simulink model "HIL_test"  (Simulink 7.5)
settings: Solver=FixedStepDiscrete  SolverMode=SingleTasking  StartTime=0.0  StopTime=10.0  FixedStep=0.01  RelTol=1e-3
undefined symbols (not defined in the file): enableHil, Function_Update, getSensorData, Init_onlyOnce, Init_Reset, initUart2, processNewCommData, y1
libraries: dsPICdrivers x7
settings Model: Creator=Bryant  LastModifiedBy=Bryant
settings OptimizationCC: OptimizeModelRefInitCode=on  LifeSpan=1
settings HardwareCC: ProdBitPerInt=16  ProdEndianess=LittleEndian  ProdWordSize=16  ProdHWDeviceType=16-bit Generic
settings RTWCC: SystemTargetFile=dspic.tlc  MakeCommand=make_CreateMPLAB  TemplateMakefile=dspic_pic30_gcc.tmf  PostCodeGenCommand=dsPIC_Compile()  Description=Embedded Target for Microchip dsPIC (real-time)  ProcessScript=dspic_make_rtw_hook
settings RTWCC: CustomSource=|
  | ../clib/circBuffer.c
  | ../clib/commProtocol.c
  | ../clib/uart2.c
settings CodeAppCC: IgnoreCustomStorageClasses=off
settings STFCustomTargetCC: IncludeMdlTerminateFcn=off  CombineOutputUpdateFcns=on  SuppressErrorStatus=on  ERTCustomFileBanners=on  SupportContinuousTime=off  SupportNonInlinedSFcns=off  SystemTargetFile=dspic.tlc
settings ERTTargetCC: MultiwordLength=2048  ParMdlRefBuildCompliant=off  CompOptLevelCompliant=off  IncludeMdlTerminateFcn=off  SuppressErrorStatus=on  ERTFirstTimeCompliant=off  ModelStepFunctionPrototypeControlCompliant=off  CPPClassGenCompliant=off  ExtModeMexFile=ext_serial_win32_comm  InlinedParameterPlacement=NonHierarchical  ERTSrcFileBannerTemplate=dsPIC_code_template.cgt  ERTHdrFileBannerTemplate=dsPIC_code_template.cgt  ERTDataSrcFileTemplate=dsPIC_code_template.cgt  ERTDataHdrFileTemplate=dsPIC_code_template.cgt  ERTCustomFileTemplate=dsPIC_main.tlc  ConvertIfToSwitch=off
settings CustomProperty: DataType=string  Value=C:\PROGRA~1\MATLAB\R2010a\bin\win64\gmake

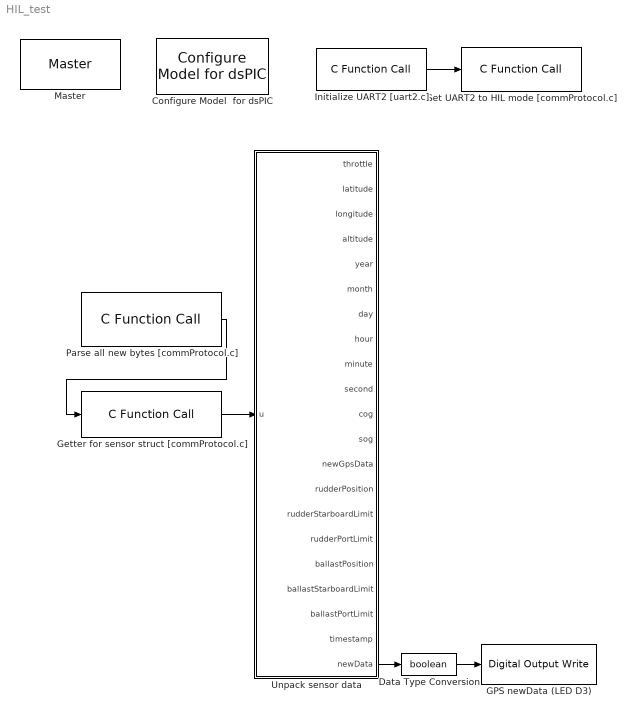
== system HIL_test ==
  Configure Model  for dsPIC : dsPICdrivers/Simulink Configuration/Configure Model  for dsPIC
  Data Type Conversion : DataTypeConversion  OutDataTypeMode=boolean  OutDataType=fixdt(1, 16)  OutScaling=2^0  OutDataTypeStr=boolean
  GPS newData (LED D3) : dsPICdrivers/Digital I//O/Digital Output Write  Tag=dsPIC_Digital_Output  Priority=5  PORT=A  Pin=[0]  Simultaneous=off  OrderingInOutPopup=None
  Getter for sensor struct [commProtocol.c] : dsPICdrivers/OTHERS/C Function Call  Tag=dsPIC_dsPIC_CFunctionCall  FctUpdate=Output Function  fctName='getSensorData'  INPUT_SIZE=1  INPUT1=--  INPUT2=--  INPUT3=--  OUTPUT_SIZE=40  OUTPUT1=uint8  SampleTime=.01  InputType=[ ]  OutputType=[ 2 ]  FctDeclaration=extern void getSensorData(uint8_T* y1);  FctCall=getSensorData(*%y1);  OrderingInOutPopup=Input  FctStart=None  FctStart_Name=Init_onlyOnce  FctStart_Declaration=inline extern void Init_onlyOnce();  FctStart_Call=Init_onlyOnce();  FctInit=None  FctInit_Name=Init_Reset  FctInit_Declaration=inline extern void Init_Reset();  FctInit_Call=Init_Reset();
  Initialize UART2 [uart2.c] : dsPICdrivers/OTHERS/C Function Call  Tag=dsPIC_dsPIC_CFunctionCall  FctUpdate=None  fctName='initUart2'  INPUT_SIZE=1  INPUT1=--  INPUT2=--  INPUT3=--  OUTPUT_SIZE=1  OUTPUT1=--  SampleTime=Inf  InputType=[]  OutputType=[]  FctDeclaration=extern void initUart2();  FctCall=initUart2();  OrderingInOutPopup=Output  FctStart=Start Function (Call once and only once)  FctStart_Name=initUart2  FctStart_Declaration=inline extern void initUart2();  FctStart_Call=initUart2();  FctInit=None  FctInit_Name=Init_Reset  FctInit_Declaration=inline extern void Init_Reset();  FctInit_Call=Init_Reset();
  Master : dsPICdrivers/Master  Tag=dsPIC_MASTER  Priority=1  TimeStepType=Timer1  picType=33fJ256GP710  fcy=40000000  Quartz_33f=8e6  PLLActive_33f=on  fcyDesired_33f=40000000  tmr1="[8  49999  0]"  tmr1Info="Time Step : 0.01  ;   Error : 0%  PR1=49999"  tmr2345="[0  0  0  0  0  0  0  0]"  tmr2345cfg=[-1 -1 -1 -1 -1 -1 -1 -1]  IOautoConf=on  typePort="[ 10   0   0   0   0   0   0   0   0   0   0   0   0   0   0   0   0   0   0   0   0   0   0   0   0   0   0   0   0   0   0   0   0   0   0   0   0   0   0   0   0   0   0   0   0   0   0   0   0   0   0   0   0   0   0   0   0   0   0   0   0   0   0   0   0   0   0   0   0   0   0   0   0   0   0   0   0   0   0   0   0   0   0   0   0   0   0   0   0   0   0   0   0   0   0   0   0   0   0   0   0   0   0   0   0   0   0   0   0   0   0   0 ]"  TRIS="[ 65534  65535  65535  65535  65535  65535  65535 ]"  ADPCFG=0  MasterBusyPort=None  MasterOverloadPort=None  FOSC=Quartz (XT - HS)  ClockSwitchMonitor=Both disabled  TempProtection_33f=TEMP_ON  FPBOR=<empty>  PWRT=disable  MCLR=<empty>  ICD=ICS_PGD1  JTAGEN=JTAGEN_OFF  PowerSave=off  OverrideFcy=off  NewFcy=1e6  PR2345="[65535  65535  65535  65535  65535  65535  65535  65535]"
  Parse all new bytes [commProtocol.c] : dsPICdrivers/OTHERS/C Function Call  Tag=dsPIC_dsPIC_CFunctionCall  FctUpdate=Output Function  fctName='processNewCommData'  INPUT_SIZE=1  INPUT1=--  INPUT2=--  INPUT3=--  OUTPUT_SIZE=1  OUTPUT1=--  SampleTime=.01  InputType=[ ]  OutputType=[ ]  FctDeclaration=extern void processNewCommData();  FctCall=processNewCommData();  OrderingInOutPopup=Output  FctStart=None  FctStart_Name=Init_onlyOnce  FctStart_Declaration=inline extern void Init_onlyOnce();  FctStart_Call=Init_onlyOnce();  FctInit=None  FctInit_Name=Init_Reset  FctInit_Declaration=inline extern void Init_Reset();  FctInit_Call=Init_Reset();
  Set UART2 to HIL mode [commProtocol.c] : dsPICdrivers/OTHERS/C Function Call  Tag=dsPIC_dsPIC_CFunctionCall  FctUpdate=None  fctName='Function_Update'  INPUT_SIZE=1  INPUT1=uint8  INPUT2=--  INPUT3=--  OUTPUT_SIZE=1  OUTPUT1=--  SampleTime=inf  InputType=[]  OutputType=[]  FctDeclaration=extern void Function_Update();  FctCall=Function_Update();  OrderingInOutPopup=Input  FctStart=Start Function (Call once and only once)  FctStart_Name='enableHil'  FctStart_Declaration=inline extern void enableHil();  FctStart_Call=enableHil();  FctInit=None  FctInit_Name=Init_Reset  FctInit_Declaration=inline extern void Init_Reset();  FctInit_Call=Init_Reset();
  Unpack sensor data : Stateflow chart  TreatAsAtomicUnit=on
  wires:
  Getter for sensor struct [commProtocol.c]/1 -> Unpack sensor data/1(u)
  Parse all new bytes [commProtocol.c]/1 -> Getter for sensor struct [commProtocol.c]/1
  Unpack sensor data/21(newData) -> Data Type Conversion/1
  Initialize UART2 [uart2.c]/1 -> Set UART2 to HIL mode [commProtocol.c]/1
  Data Type Conversion/1 -> GPS newData (LED D3)/1

== matlab function Unpack sensor data ==
  data: u input uint8; throttle output double; latitude output double; longitude output double; altitude output double; year output double; month output double; day output double; hour output double; minute output double; second output double; cog output double; sog output double; newGpsData output double; rudderPosition output double; rudderStarboardLimit output double; rudderPortLimit output double; ballastPosition output double; ballastStarboardLimit output double; ballastPortLimit output double; timestamp output double; newData output uint8
function [throttle, latitude, longitude, altitude, year, month, day, hour, minute, second, cog, sog, newGpsData, rudderPosition, rudderStarboardLimit, rudderPortLimit, ballastPosition, ballastStarboardLimit, ballastPortLimit, timestamp, newData] = unpack(u)
%#eml

throttle = typecast(u(1:2), 'int16');
latitude = typecast(u(3:6), 'single');
longitude = typecast(u(7:10), 'single');
altitude = typecast(u(11:14), 'single');
year = u(15);
month = u(16);
day = u(17);
hour = u(18);
minute = u(19);
second = u(20);
cog = typecast(u(21:24), 'single');
sog = typecast(u(25:28), 'single');
newGpsData = u(29);
rudderPosition = typecast(u(30:31), 'uint16');
rudderStarboardLimit = u(32);
rudderPortLimit = u(33);
ballastPosition = typecast(u(34:35), 'uint16');
ballastStarboardLimit = u(36);
ballastPortLimit = u(37);
timestamp = typecast(u(38:39), 'int16');
newData = u(40);
